simulink model "QIP"  (R2019a)
settings: Solver=VariableStepAuto  StartTime=0.0  StopTime=simulationStopTime  MaxStep=0.05  RelTol=1e-3
values from neighbouring files (symbols this model uses):
  IMAX_UPM = 3    [setup.m]
  impulse_data = [50, 0.005, 1]    [setup.m]
  Mc = Mc + Eff_g * Kg^2 * Jm / r_mp^2    [setup.m]
  VMAX_DAC = 10    [setup.m]
undefined symbols (not defined in the file or in its folder): Beq, Bp, ctf_den, ctf_num, Eff_g, Eff_m, g, Ip, Kg, Km, Kt, Lp, lp, Mp, r_mp, Rm, X, Y, Z
libraries: sm_lib x33, nesl_utility x5
(part 2 of 2)

== matlab function QIP/MATLAB Function ==
  data: nxt_xduck output; xduck input; t input; fd output; impulse_data input
 function [nxt_xduck, fd]   = angle_impulse( xduck, t, impulse_data)

% This function adds a short angular acceleration fd (rad/s/s) into the
% equations of motion. 

% It also calculates the position of the impulse duck solid over time. 
% Previous position: xduck, Next position: nxt_xduck

% Global Variables needed from user: tdur, tstart fmag 
% known as impulse_duration, impulse_start, impulse_magnitude

% impulse is a rectangular pulse of magnitude fmag with period tdur
% occuring at tstart 
tdur =impulse_data(2);
fmag = -impulse_data(1);
tstart = impulse_data(3);

% Apply impulse: 
if t > 0.9*tstart && t < 0.9*tstart + tdur
    fd =  - fmag;
else
    fd = 0;
end

% Calculate duck position (apply animation):
xduck_0 = 0.3; % initial duck position 

if t >= 0.9*tstart && t <= 0.9*tstart + 10*tdur  
    nxt_xduck = xduck_0  - xduck_0 * exp(20*(t-0.9*tstart));
    if abs(xduck) >= 10
        nxt_xduck = 1* xduck;
    end
elseif t > 0.9*tstart + tdur
    nxt_xduck = xduck_0 * (1- exp(-5*(t-(0.9*tstart + tdur)))*cos(10*t));
else 
    nxt_xduck = xduck_0  + 0.05 * cos(10*t*t);
end


end
